simulink model "simulunk3"  (R2016a)
settings: Solver=VariableStepAuto  StartTime=0.0  StopTime=20  RelTol=1e-3
libraries: dspsrcs4 x1
settings Model: Creator=user  LastModifiedBy=user

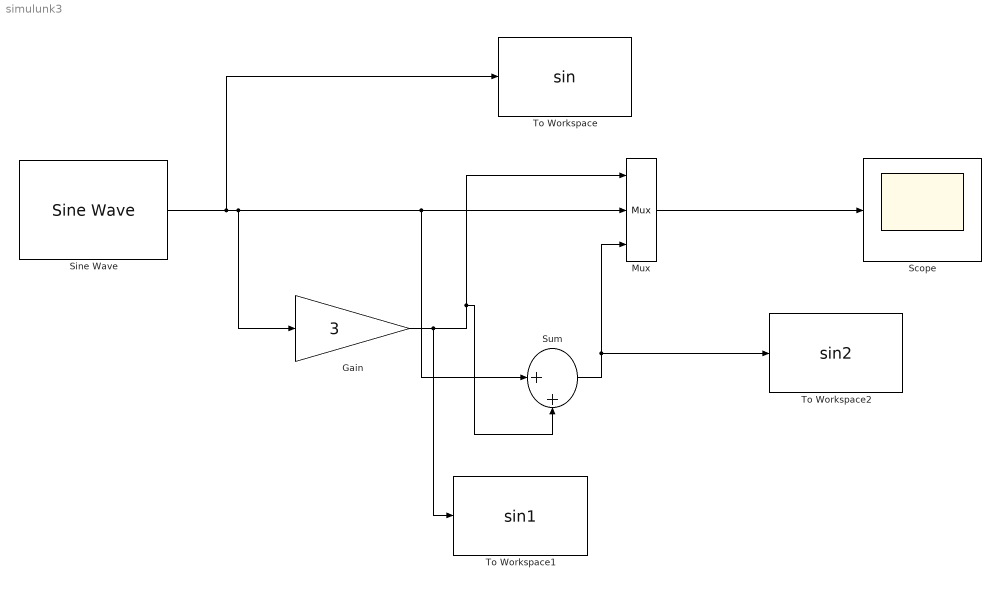
== system simulunk3 ==
  Gain : Gain  Gain=3
  Mux : Mux  Inputs=3
  Scope : Scope
  Sine Wave : dspsrcs4/Sine Wave  Amplitude=5  Frequency=1454  Phase=0  SampleMode=Continuous  OutComplex=Complex  CompMethod=Trigonometric fcn  TableSize=Speed  SampleTime=1/1000  SamplesPerFrame=1  ResetState=Restart at time zero  OutputFrames=off  dataType=double  wordLen=16  udDataType=sfix(16)  fracBitsMode=Best precision  numFracBits=15  OutDataTypeStr=double  LastOutDataTypeStr=double
  Sum : Sum  Inputs=|++
  To Workspace : ToWorkspace  VariableName=sin  SampleTime=-1
  To Workspace1 : ToWorkspace  VariableName=sin1  SampleTime=-1
  To Workspace2 : ToWorkspace  VariableName=sin2  SampleTime=-1
  wires:
  Mux/1 -> Scope/1
  Sine Wave/1 -> To Workspace/1, Gain/1, Sum/1, Mux/2
  Gain/1 -> To Workspace1/1, Sum/2, Mux/1
  Sum/1 -> Mux/3, To Workspace2/1
